simulink model "full_simulation_split_hil_new_connection"  (Simulink 7.9)
settings: Solver=ode1  StartTime=0  StopTime=10  FixedStep=Ts  RelTol=1e-8
values from neighbouring files (symbols this model uses):
  A_fx = 2e-2 * 0.4    (= 0.008)    [QR_DI_Init.m]    (also in quadro_cascade_disturbance_wo_wind.m)
  A_fy = A_fx    (= 0.008)    [QR_DI_Init.m]    (also in quadro_cascade_disturbance_wo_wind.m)
  A_fz = 2 * A_fx    (= 0.016)    [QR_DI_Init.m]    (also in quadro_cascade_disturbance_wo_wind.m)
  Bias_Phi = -0.0088    [QR_DI_Init.m]    (also in Reference_Calibration.m = mean(Phi))
  Bias_Theta = 0.022    [QR_DI_Init.m]    (also in Reference_Calibration.m = mean(Theta))
  command_on = 1    [QR_DI_Init.m]    (also in quadro_cascade_disturbance_wo_wind.m)
  cw_x = 1.05    [QR_DI_Init.m]    (also in quadro_cascade_disturbance_wo_wind.m)
  cw_y = cw_x    (= 1.05)    [QR_DI_Init.m]    (also in quadro_cascade_disturbance_wo_wind.m)
  cw_z = 1.05    [QR_DI_Init.m]    (also in quadro_cascade_disturbance_wo_wind.m)
  deltaTm = 0.2    [QR_DI_Init.m]    (also in quadro_cascade_disturbance_wo_wind.m)
  den_psi_ref = poly( ones(1,2) * -1 * T_psi_ref)    [QR_DI_Init.m]    (also in quadro_cascade_disturbance_wo_wind.m)
  den_x_ref = poly( ones(1,4) * -1 * T_x_ref)    [QR_DI_Init.m]    (also in quadro_cascade_disturbance_wo_wind.m)
  den_y_ref = poly( ones(1,4) * -1 * T_y_ref)    [QR_DI_Init.m]    (also in quadro_cascade_disturbance_wo_wind.m)
  den_z_ref = poly( ones(1,4) * -1 * T_z_ref)    [QR_DI_Init.m]    (also in quadro_cascade_disturbance_wo_wind.m)
  drot = 0.0117    [QR_DI_Init.m]    (also in quadro_cascade_disturbance_wo_wind.m = 0.2)
  dtran = 0.01    [QR_DI_Init.m]    (also in quadro_cascade_disturbance_wo_wind.m = 0.003)
  Fz_gain = 1 + 0.05*rand(1)    [QR_DI_Init.m]    (also in quadro_cascade_disturbance_wo_wind.m)
  Fz_lo = - 1.2 * m * g    (= -3.5316)    [QR_DI_Init.m]    (also in quadro_cascade_disturbance_wo_wind.m = -4.1202)
  Fz_up = 0    [QR_DI_Init.m]    (also in quadro_cascade_disturbance_wo_wind.m)
  g = 9.81    [QR_DI_Init.m]    (also in quadro_cascade_disturbance_wo_wind.m)
  Iq = [I_xx 0 0 ; 0 I_yy 0 ; 0 0 I_zz ]    [QR_DI_Init.m]    (also in quadro_cascade_disturbance_wo_wind.m = [0.0605 0 0; 0 0.0605 0; 0 0 0.018])
  K_err = old(:,2:end)    [QR_DI_Init.m]    (also in quadro_cascade_disturbance_wo_wind.m)
  K_Mot_Force = 0.3512    [QR_DI_Init.m]    (also in quadro_cascade_disturbance_wo_wind.m)
  K_Mot_Torque = 0.013    [QR_DI_Init.m]    (also in quadro_cascade_disturbance_wo_wind.m = 0.0013)
  l = 0.25    [QR_DI_Init.m]    (also in quadro_cascade_disturbance_wo_wind.m = 0.2775)
  m = 0.30    (= 0.3)    [QR_DI_Init.m]    (also in quadro_cascade_disturbance_wo_wind.m)
  m_real = m * ( 1 + 0.05*rand(1))    [QR_DI_Init.m]    (also in quadro_cascade_disturbance_wo_wind.m)
  Mm = 0.0    (= 0)    [QR_DI_Init.m]    (also in quadro_cascade_disturbance_wo_wind.m = 0.5)
  Mx_lo = - Mx_up    (= -0.2)    [QR_DI_Init.m]    (also in quadro_cascade_disturbance_wo_wind.m)
  Mx_up = 0.20    (= 0.2)    [QR_DI_Init.m]    (also in quadro_cascade_disturbance_wo_wind.m)
  My_lo = - My_up    (= -0.2)    [QR_DI_Init.m]    (also in quadro_cascade_disturbance_wo_wind.m)
  My_up = 0.20    (= 0.2)    [QR_DI_Init.m]    (also in quadro_cascade_disturbance_wo_wind.m)
  Mz_lo = - Mz_up    (= -0.02)    [QR_DI_Init.m]    (also in quadro_cascade_disturbance_wo_wind.m = -0.002)
  Mz_up = 0.02    [QR_DI_Init.m]    (also in quadro_cascade_disturbance_wo_wind.m = 0.002)
  phase_wind_z = 0    [QR_DI_Init.m]    (also in quadro_cascade_disturbance_wo_wind.m)
  psi_p_lim = 10*pi/180    (= 0.174532925199)    [QR_DI_Init.m]    (also in quadro_cascade_disturbance_wo_wind.m = 5)
  PWM_MAX = 200    [QR_DI_Init.m]    (also in quadro_cascade_disturbance_wo_wind.m)
  rho_air = 1.2041    [QR_DI_Init.m]    (also in quadro_cascade_disturbance_wo_wind.m)
  sample_time_noise_psi = 0.1    [QR_DI_Init.m]
  sample_time_noise_x = 0.2    [QR_DI_Init.m]
  sample_time_noise_y = 0.2    [QR_DI_Init.m]
  sample_time_noise_z = 0.1    [QR_DI_Init.m]
  seed_psi = seedvector(7)    [QR_DI_Init.m]
  seed_x = seedvector(1)    [QR_DI_Init.m]    (also in quadro_cascade_disturbance_wo_wind.m)
  seed_xp = seedvector(4)    [QR_DI_Init.m]    (also in quadro_cascade_disturbance_wo_wind.m)
  seed_y = seedvector(2)    [QR_DI_Init.m]    (also in quadro_cascade_disturbance_wo_wind.m)
  seed_yp = seedvector(5)    [QR_DI_Init.m]    (also in quadro_cascade_disturbance_wo_wind.m)
  seed_z = seedvector(3)    [QR_DI_Init.m]    (also in quadro_cascade_disturbance_wo_wind.m)
  seed_zp = seedvector(6)    [QR_DI_Init.m]    (also in quadro_cascade_disturbance_wo_wind.m)
  std_dev_psi = 1 * pi/180 * Noise_on    (= 0)    [QR_DI_Init.m]
  std_dev_x = 1e-1 * Noise_on    (= 0)    [QR_DI_Init.m]
  std_dev_xp = 0.03 * Noise_on    (= 0)    [QR_DI_Init.m]
  std_dev_y = 1e-1 * Noise_on    (= 0)    [QR_DI_Init.m]
  std_dev_yp = 0.03 * Noise_on    (= 0)    [QR_DI_Init.m]
  std_dev_z = 0.03 * Noise_on    (= 0)    [QR_DI_Init.m]
  std_dev_zp = 0.03 * Noise_on    (= 0)    [QR_DI_Init.m]
  T_refalt = 0.01    [QR_DI_Init.m]    (also in quadro_cascade_disturbance_wo_wind.m)
  T_wind_z = 24    [QR_DI_Init.m]    (also in quadro_cascade_disturbance_wo_wind.m)
  Tm = 10    [QR_DI_Init.m]    (also in quadro_cascade_disturbance_wo_wind.m)
  Ts = 1e-2    (= 0.01)    [QR_DI_Init.m]    (also in quadro_cascade_disturbance_wo_wind.m)
  v_wind_max_z = 2    [QR_DI_Init.m]    (also in quadro_cascade_disturbance_wo_wind.m)
  wind_on = 0    [QR_DI_Init.m]    (also in quadro_cascade_disturbance_wo_wind.m)
  x_p_lim = 1.5    [QR_DI_Init.m]    (also in quadro_cascade_disturbance_wo_wind.m = 5)
  y_p_lim = 1.5    [QR_DI_Init.m]    (also in quadro_cascade_disturbance_wo_wind.m = 5)
  z_p_lim = 1    [QR_DI_Init.m]    (also in quadro_cascade_disturbance_wo_wind.m = 1.5)
undefined symbols (not defined in the file or in its folder): T_wind_fine, v_wind_x_fine, v_wind_y_fine
libraries: simulink x5, dspsigops x4, Ports x4, aerolibtransform2 x3, dspmtrx3 x1, aerolibutil x1
(part 1 of 6)
settings Model: Creator=Richard  LastModifiedBy=uav  SimulationMode=accelerator  ExtModeTrigDuration=100
settings OptimizationCC: InitFltsAndDblsToZero=on
settings DebuggingCC: FcnCallInpInsideContextMsg=Use local settings  StrictBusMsg=Warning
settings HardwareCC: ProdIntDivRoundTo=Zero  ProdEndianess=LittleEndian  ProdHWDeviceType=Intel->x86/Pentium  TargetBitPerLong=64  TargetBitPerPointer=64  TargetEndianess=LittleEndian  TargetWordSize=64  TargetHWDeviceType=MATLAB Host  ProdEqTarget=off
settings RTWCC: SystemTargetFile=orocos.tlc  TemplateMakefile=orocos.tmf  Description=Linux Orocos Target  RTWVerbose=off  ProcessScript=orocos_make_rtw_hook
settings CodeAppCC: GenerateComments=off  MaxIdLength=128  SimulinkBlockComments=off
settings STFCustomTargetCC: CodeReplacementLibrary=ANSI_C  ModelReferenceCompliant=off  GeneratePreprocessorConditionals=Disable all  MatFileLogging=on  SystemTargetFile=orocos.tlc

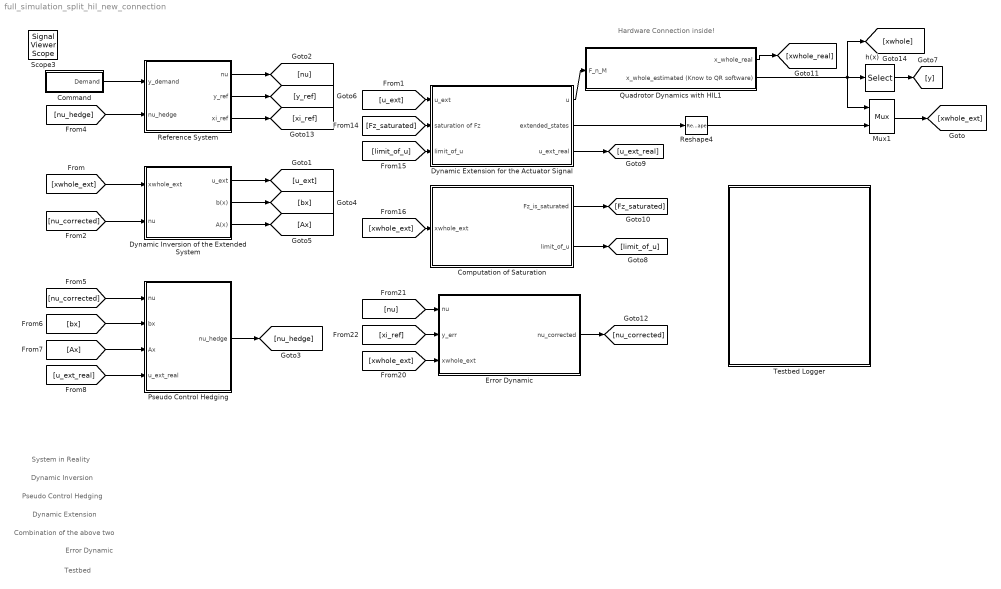
== system full_simulation_split_hil_new_connection ==
  note: System in Reality
  note: Dynamic Extension
  note: Dynamic Inversion
  note: Pseudo Control Hedging
  note: Combination of the above two
  note: Error Dynamic
  note: Testbed
  note: Hardware Connection inside!
  Command : Subsystem
  Computation of Saturation : Subsystem
  Dynamic Extension for the Actuator Signal : Subsystem
  Dynamic Inversion of the Extended System : Subsystem
  Error Dynamic : Subsystem
  Mux1 : Mux  Inputs=2
  Pseudo Control Hedging : Subsystem
  Quadrotor Dynamics with HIL1 : Subsystem
  Reference System : Subsystem
  Reshape4 : Reshape  OutputDimensionality=Column vector (2-D)  OutputDimensions=[1:3]
  Testbed Logger : Subsystem
  h(x) : Selector  InputPortWidth=12  IndexOptions=Index vector (dialog)  Indices=[1 2 3 9]  OutputSizes=1
  Scope3 : SignalViewerScope  IOType=viewer  NumInputPorts=4  RefreshTime=0.035000
  wires:
  Reference System/1(nu) -> [nu]
  Dynamic Extension for the Actuator Signal/1(u) -> Quadrotor Dynamics with HIL1/1(F_n_M)
  Quadrotor Dynamics with HIL1/2(x_whole_estimated (Know to QR software)) -> h(x)/1, [xwhole], Mux1/1
  Dynamic Extension for the Actuator Signal/2(extended_states) -> Reshape4/1
  Dynamic Inversion of the Extended System/1(u_ext) -> [u_ext]
  Mux1/1 -> [xwhole_ext]
  [u_ext] -> Dynamic Extension for the Actuator Signal/1(u_ext)
  Reshape4/1 -> Mux1/2
  h(x)/1 -> [y]
  [nu_hedge] -> Reference System/2(nu_hedge)
  [xwhole_ext] -> Dynamic Inversion of the Extended System/1(xwhole_ext)
  [nu_corrected] -> Dynamic Inversion of the Extended System/2(nu)
  Dynamic Inversion of the Extended System/2(b(x)) -> [bx]
  Dynamic Inversion of the Extended System/3(A(x)) -> [Ax]
  [nu_corrected] -> Pseudo Control Hedging/1(nu)
  [bx] -> Pseudo Control Hedging/2(bx)
  [Ax] -> Pseudo Control Hedging/3(Ax)
  [u_ext_real] -> Pseudo Control Hedging/4(u_ext_real)
  Reference System/2(y_ref) -> [y_ref]
  Pseudo Control Hedging/1(nu_hedge) -> [nu_hedge]
  [Fz_saturated] -> Dynamic Extension for the Actuator Signal/2(saturation of Fz)
  Dynamic Extension for the Actuator Signal/3(u_ext_real) -> [u_ext_real]
  Computation of Saturation/2(limit_of_u) -> [limit_of_u]
  [limit_of_u] -> Dynamic Extension for the Actuator Signal/3(limit_of_u)
  [xwhole_ext] -> Computation of Saturation/1(xwhole_ext)
  Computation of Saturation/1(Fz_is_saturated) -> [Fz_saturated]
  Reference System/3(xi_ref) -> [xi_ref]
  [nu] -> Error Dynamic/1(nu)
  [xi_ref] -> Error Dynamic/2(y_err)
  [xwhole_ext] -> Error Dynamic/3(xwhole_ext)
  Error Dynamic/1(nu_corrected) -> [nu_corrected]
  Command/1(Demand) -> Reference System/1(y_demand)
  Quadrotor Dynamics with HIL1/1(x_whole_real) -> [xwhole_real]

== system full_simulation_split_hil_new_connection/Command ==
  CommandOn : Gain  Gain=command_on
  From Workspace : FromWorkspace  VariableName=Mission_Outdoor_steps  SampleTime=0  Interpolate=off  OutputAfterFinalValue=Holding final value
  From Workspace1 : FromWorkspace  VariableName=Mission_Indoor_steps  SampleTime=0  Interpolate=off  OutputAfterFinalValue=Holding final value
  Step 1 : Step  Time=75  Before=zeros(1,4)  After=[25 15 -25 20*pi/180]*1  SampleTime=0
  Step 2 : Step  Time=100  Before=zeros(1,4)  After=[-24 -24 20 -40*pi/180]*1  SampleTime=0
  Step 3 : Step  Time=15  Before=zeros(1,4)  After=[50 50 50 0]*1  SampleTime=0
  Sum2 : Sum  Inputs=2
  Demand : Outport
  wires:
  Sum2/1 -> CommandOn/1
  CommandOn/1 -> Demand/1
  From Workspace/1 -> Sum2/1

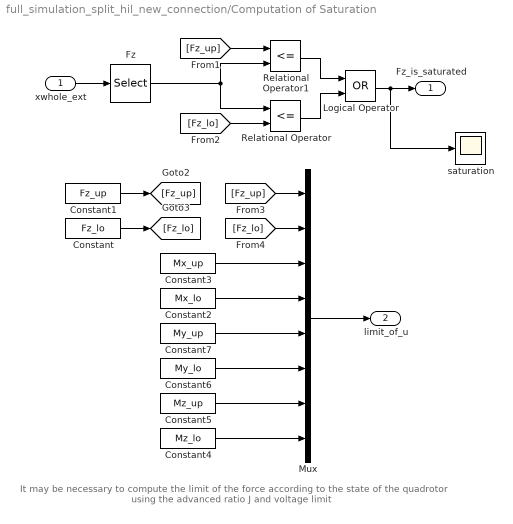
== system full_simulation_split_hil_new_connection/Computation of Saturation ==
  note: It may be necessary to compute the limit of the force according to
      | the state of the quadrotor using the advanced ratio J and voltage limit
  xwhole_ext : Inport
  Constant : Constant  Value=Fz_lo
  Constant1 : Constant  Value=Fz_up
  Constant2 : Constant  Value=Mx_lo
  Constant3 : Constant  Value=Mx_up
  Constant4 : Constant  Value=Mz_lo
  Constant5 : Constant  Value=Mz_up
  Constant6 : Constant  Value=My_lo
  Constant7 : Constant  Value=My_up
  Fz : Selector  InputPortWidth=14  IndexOptions=Index vector (dialog)  Indices=[13]  OutputSizes=1
  Logical Operator : Logic  Operator=OR  AllPortsSameDT=off  OutDataTypeStr=boolean
  Mux : Mux  Inputs=8
  Relational Operator : RelationalOperator  Operator=<=  OutDataTypeStr=boolean
  Relational Operator1 : RelationalOperator  Operator=<=  OutDataTypeStr=boolean
  saturation : Scope
      settings: YMin=-27.5  YMax=27.5  SaveName=ScopeData11
  Fz_is_saturated : Outport
  limit_of_u : Outport  Port=2
  wires:
  xwhole_ext/1 -> Fz/1
  [Fz_up] -> Mux/1
  [Fz_lo] -> Mux/2
  Constant1/1 -> [Fz_up]
  Constant/1 -> [Fz_lo]
  Constant3/1 -> Mux/3
  Constant4/1 -> Mux/8
  Constant2/1 -> Mux/4
  Constant7/1 -> Mux/5
  Constant6/1 -> Mux/6
  Constant5/1 -> Mux/7
  [Fz_up] -> Relational Operator1/1
  Relational Operator1/1 -> Logical Operator/1
  Relational Operator/1 -> Logical Operator/2
  Logical Operator/1 -> Fz_is_saturated/1, saturation/1
  Mux/1 -> limit_of_u/1
  [Fz_lo] -> Relational Operator/2
  Fz/1 -> Relational Operator1/2, Relational Operator/1

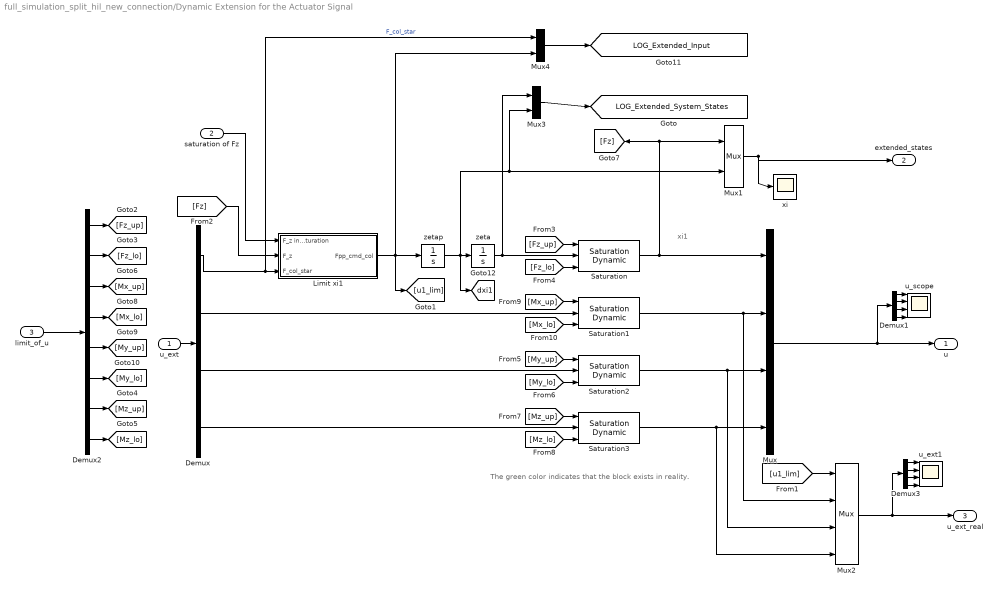
== system full_simulation_split_hil_new_connection/Dynamic Extension for the Actuator Signal ==
  note: xi1
  note: The green color indicates that the
      | block exists in reality.
  u_ext : Inport
  saturation of Fz : Inport  Port=2
  limit_of_u : Inport  Port=3
  Demux : Demux
  Demux1 : Demux
  Demux2 : Demux  Outputs=8
  Demux3 : Demux
  Limit xi1 : Subsystem
  Mux : Mux
  Mux1 : Mux  Inputs=2
  Mux2 : Mux
  Mux3 : Mux  Inputs=2
  Mux4 : Mux  Inputs=2
  Saturation{,1..3} (4 alike) : simulink/Discontinuities/Saturation Dynamic  OutMin=[]  OutMax=[]  OutDataTypeStr=Inherit: Same as second input  OutDataType=sfix(16)  OutScaling=2^-10  DoSatur=off
  u_ext1 : Scope  NumInputPorts=4
      settings: TimeRange=1  YMin=0~0~0~-5  YMax=1~1~1~5  SaveName=ScopeData9
  u_scope : Scope  NumInputPorts=4
      settings: TimeRange=40  YMin=8~-6~-15~-8  YMax=20~8~10~4  SaveName=ScopeData12
  xi : Scope
      settings: YMin=-27.5  YMax=27.5  SaveName=ScopeData7
  zeta : Integrator
  zetap : Integrator
  u : Outport
  extended_states : Outport  Port=2
  u_ext_real : Outport  Port=3
  tag scope: LOG_Extended_Input=global, LOG_Extended_System_States=global, dxi1=global
  wires:
  u_ext/1 -> Demux/1
  Demux/2 -> Saturation1/2
  Demux/3 -> Saturation2/2
  Demux/4 -> Saturation3/2
  zeta/1 -> Saturation/2, Mux3/1
  Mux1/1 -> extended_states/1, xi/1
  Demux1/1 -> u_scope/1
  Demux1/2 -> u_scope/2
  Demux1/3 -> u_scope/3
  Demux1/4 -> u_scope/4
  saturation of Fz/1 -> Limit xi1/1(F_z in saturation)
  Mux2/1 -> u_ext_real/1, Demux3/1
  Demux/1 -> Limit xi1/3(F_col_star), Mux4/1  "F_col_star"
  [Fz] -> Limit xi1/2(F_z)
  Saturation/1 -> Mux/1, Mux1/1, [Fz]
  Saturation1/1 -> Mux/2, Mux2/2
  Saturation2/1 -> Mux/3, Mux2/3
  Saturation3/1 -> Mux/4, Mux2/4
  Mux/1 -> u/1, Demux1/1
  [u1_lim] -> Mux2/1
  [Fz_up] -> Saturation/1
  [Fz_lo] -> Saturation/3
  [Mz_up] -> Saturation3/1
  [Mz_lo] -> Saturation3/3
  [Mx_up] -> Saturation1/1
  [Mx_lo] -> Saturation1/3
  [My_up] -> Saturation2/1
  [My_lo] -> Saturation2/3
  Demux2/1 -> [Fz_up]
  Demux2/2 -> [Fz_lo]
  Demux2/3 -> [Mx_up]
  Demux2/4 -> [Mx_lo]
  Demux2/5 -> [My_up]
  Demux2/6 -> [My_lo]
  Demux2/7 -> [Mz_up]
  Demux2/8 -> [Mz_lo]
  limit_of_u/1 -> Demux2/1
  Demux3/1 -> u_ext1/1
  Demux3/2 -> u_ext1/2
  Demux3/3 -> u_ext1/3
  Demux3/4 -> u_ext1/4
  Limit xi1/1(Fpp_cmd_col) -> [u1_lim], zetap/1, Mux4/2
  zetap/1 -> [dxi1], zeta/1, Mux1/2, Mux3/2
  Mux3/1 -> [LOG_Extended_System_States]
  Mux4/1 -> [LOG_Extended_Input]

== system full_simulation_split_hil_new_connection/Dynamic Inversion of the Extended System ==
  xwhole_ext : Inport
  nu : Inport  Port=2
  Add2 : Sum
  Ber. alpha(x) : Subsystem
  Ber. beta(x) : Subsystem
  Divide1 : Product  Inputs=**  Multiplication=Matrix(*)
  bx SH : Subsystem  mask{m=m, Iq=Iq, dtran=dtran, drot=drot}
      mask prompts: m "Mass"; Iq "Inertia"; dtran "Translational Damping Constan"; drot "Rotational Damping Constant"
  bx1 : Subsystem  mask{m=m, Iq=Iq, dtran=dtran, drot=drot}
      mask prompts: m "Mass"; Iq "Inertia"; dtran "Translational Damping Constan"; drot "Rotational Damping Constant"
  invAx SH : Subsystem  mask{m=m, Iq=Iq, dtran=dtran, drot=drot}
      mask prompts: m "Mass"; Iq "Inertia"; dtran "Translational Damping Constan"; drot "Rotational Damping Constant"
  invAx1 : Subsystem  mask{m=m, Iq=Iq, dtran=dtran, drot=drot}
      mask prompts: m "Mass"; Iq "Inertia"; dtran "Translational Damping Constan"; drot "Rotational Damping Constant"
  u_ext : Outport
  b(x) : Outport  Port=2
  A(x) : Outport  Port=3
  wires:
  Divide1/1 -> Add2/1
  Ber. alpha(x)/1(alpha (x)) -> Add2/2
  Ber. beta(x)/1(beta (x)) -> Divide1/1
  nu/1 -> Divide1/2
  bx SH/1(bx) -> Ber. alpha(x)/2(b (x)), b(x)/1  "b(x)"
  xwhole_ext/1 -> invAx SH/1(xwhole_ext), bx SH/1(xwhole_ext)
  invAx SH/1(invAx) -> Ber. beta(x)/1(A_inv(x)), Ber. alpha(x)/1(A_inv(x))
  Add2/1 -> u_ext/1
  invAx SH/2(A(x)) -> A(x)/1

== system full_simulation_split_hil_new_connection/Error Dynamic ==
  nu : Inport
  y_err : Inport  Port=2
  xwhole_ext : Inport  Port=3
  K_err*u : Gain  Gain=K_err  Multiplication=Matrix(K*u) (u vector)
  Sum1 : Sum  Inputs=+-|
  Sum2 : Sum  Inputs=++|
  add inegratorl1 : Subsystem
  add inegratorl2 : Subsystem
  coordinate transformation1 : Subsystem  mask{m=m, Iq=Iq, dtran=dtran, drot=drot}
      mask prompts: m "Mass"; Iq "Inertia"; dtran "Translational Damping Constan"; drot "Rotational Damping Constant"
  nu_corrected : Outport
  tag scope: LOG_External_Dynamics_State_Vector=global, LOG_Reference_Input=global
  wires:
  coordinate transformation1/1(xi) -> add inegratorl1/1(In1), [LOG_External_Dynamics_State_Vector]
  Sum1/1 -> K_err*u/1
  y_err/1 -> add inegratorl2/1(In1)
  nu/1 -> Sum2/1
  Sum2/1 -> nu_corrected/1, [LOG_Reference_Input]
  xwhole_ext/1 -> coordinate transformation1/1(xwhole_ext)
  K_err*u/1 -> Sum2/2
  add inegratorl1/1(Out1) -> Sum1/2
  add inegratorl2/1(Out1) -> Sum1/1

== system full_simulation_split_hil_new_connection/Pseudo Control Hedging ==
  nu : Inport
  bx : Inport  Port=2
  Ax : Inport  Port=3
  u_ext_real : Inport  Port=4
  Add4 : Sum  Inputs=+-
  Divide4 : Product  Inputs=**  Multiplication=Matrix(*)
  nu_hat : Sum
  nu_hedge : Outport
  tag scope: LOG_Estimated_Sys_Output=global, LOG_Hedge_Signal_Vector=global
  wires:
  Divide4/1 -> nu_hat/2
  nu_hat/1 -> Add4/2, [LOG_Estimated_Sys_Output]
  nu/1 -> Add4/1
  Add4/1 -> nu_hedge/1, [LOG_Hedge_Signal_Vector]
  bx/1 -> nu_hat/1
  Ax/1 -> Divide4/1
  u_ext_real/1 -> Divide4/2

== system full_simulation_split_hil_new_connection/Quadrotor Dynamics with HIL1 ==
  note: Real: simulated reality, no noise
      | IMU: IMU from QR
  F_n_M : Inport
  Data Fusion : Subsystem
  Fz_cmd : Selector  InputPortWidth=4  IndexOptions=Index vector (dialog)  Indices=[1]  OutputSizes=1
  M_cmd : Selector  InputPortWidth=4  IndexOptions=Index vector (dialog)  Indices=[2:4]  OutputSizes=1
  Sensor Model : Subsystem
  Simulated Reality : Subsystem
  x_whole_real : Outport
  x_whole_estimated (Know to QR software) : Outport  Port=2
  tag scope: LOG_Input_Vector=global, LOG_State_Vector=global
  wires:
  M_cmd/1 -> Simulated Reality/2(M_b)
  Fz_cmd/1 -> Simulated Reality/1(F_z(b))
  Simulated Reality/2(x_whole_real) -> x_whole_real/1, Sensor Model/1(x_whole_real)
  Data Fusion/1(x_whole_estimated) -> x_whole_estimated (Know to QR software)/1, [LOG_State_Vector]
  Sensor Model/3(Yaw Angle) -> Data Fusion/4(Psi)  "Psi"
  Sensor Model/1(x_vec (Position)) -> Data Fusion/2(x_Vector)
  Sensor Model/2(xp_vec (Velocity)) -> Data Fusion/3(xp_Vector)
  Simulated Reality/1("x_angular_IMU (x_Euler, Omega)") -> Data Fusion/1("x_Euler, Omega")
  F_n_M/1 -> Fz_cmd/1, M_cmd/1, [LOG_Input_Vector]

== system full_simulation_split_hil_new_connection/Reference System ==
  y_demand : Inport
  nu_hedge : Inport  Port=2
  Rate Limiter : RateLimiter  RisingSlewLimit=[ x_p_lim y_p_lim z_p_lim psi_p_lim ]  FallingSlewLimit=- [ x_p_lim y_p_lim z_p_lim psi_p_lim ]  SampleTimeMode=inherited
  Reference System : Subsystem
  nu : Outport
  y_ref : Outport  Port=2
  xi_ref : Outport  Port=3
  tag scope: LOG_Demand=global, LOG_Reference_Sys_Output=global
  wires:
  y_demand/1 -> Rate Limiter/1, [LOG_Demand]
  Reference System/1(nu) -> nu/1, [LOG_Reference_Sys_Output]
  Reference System/2(y_ref) -> y_ref/1
  Reference System/3(xi_ref) -> xi_ref/1
  nu_hedge/1 -> Reference System/2(nu_hedge)
  Rate Limiter/1 -> Reference System/1(command)

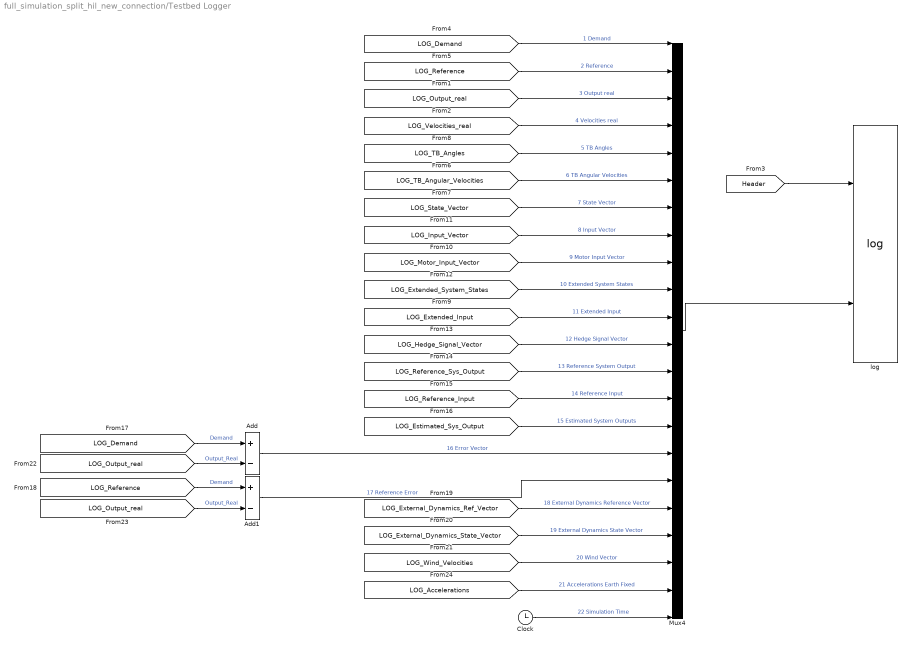
== system full_simulation_split_hil_new_connection/Testbed Logger ==
  Add : Sum  Inputs=+-
  Add1 : Sum  Inputs=+-
  Clock : Clock
  Mux4 : Mux  Inputs=22
  log : Ports/log
  wires:
  [Header] -> log/1
  Mux4/1 -> log/2
  [LOG_Demand] -> Mux4/1  "1 Demand"
  [LOG_Reference] -> Mux4/2  "2 Reference"
  [LOG_Output_real] -> Mux4/3  "3 Output real"
  [LOG_Velocities_real] -> Mux4/4  "4 Velocities real"
  [LOG_TB_Angles] -> Mux4/5  "5 TB Angles"
  [LOG_TB_Angular_Velocities] -> Mux4/6  "6 TB Angular Velocities"
  [LOG_State_Vector] -> Mux4/7  "7 State Vector"
  [LOG_Input_Vector] -> Mux4/8  "8 Input Vector"
  [LOG_Motor_Input_Vector] -> Mux4/9  "9 Motor Input Vector"
  [LOG_Extended_System_States] -> Mux4/10  "10 Extended System States"
  [LOG_Extended_Input] -> Mux4/11  "11 Extended Input"
  [LOG_Hedge_Signal_Vector] -> Mux4/12  "12 Hedge Signal Vector"
  [LOG_Reference_Sys_Output] -> Mux4/13  "13 Reference System Output"
  [LOG_Reference_Input] -> Mux4/14  "14 Reference Input"
  [LOG_Estimated_Sys_Output] -> Mux4/15  "15 Estimated System Outputs"
  Add/1 -> Mux4/16  "16 Error Vector"
  Add1/1 -> Mux4/17  "17 Reference Error"
  [LOG_External_Dynamics_Ref_Vector] -> Mux4/18  "18 External Dynamics Reference Vector"
  [LOG_External_Dynamics_State_Vector] -> Mux4/19  "19 External Dynamics State Vector"
  [LOG_Wind_Velocities] -> Mux4/20  "20 Wind Vector"
  [LOG_Demand] -> Add/1  "Demand"
  [LOG_Output_real] -> Add/2  "Output_Real"
  [LOG_Reference] -> Add1/1  "Demand"
  [LOG_Output_real] -> Add1/2  "Output_Real"
  [LOG_Accelerations] -> Mux4/21  "21 Accelerations Earth Fixed"
  Clock/1 -> Mux4/22  "22 Simulation Time"

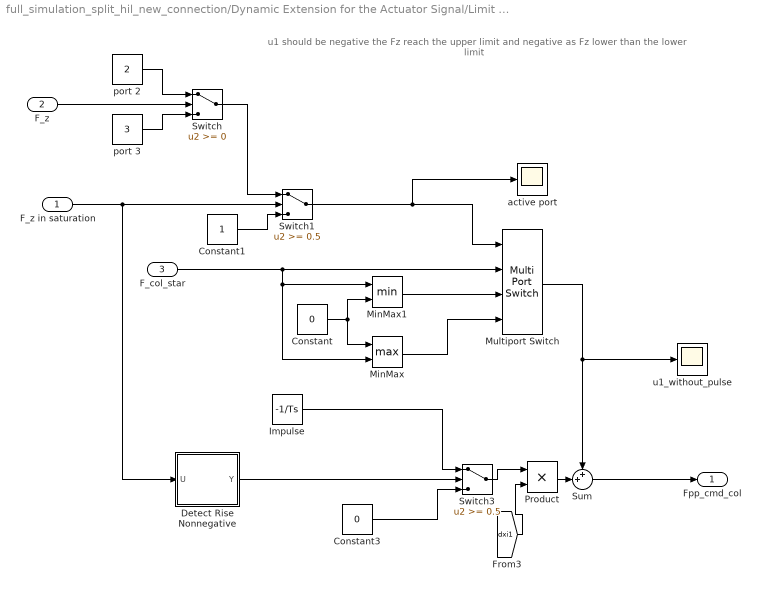
== system full_simulation_split_hil_new_connection/Dynamic Extension for the Actuator Signal/Limit xi1 ==
  note: u1 should be negative the Fz reach the upper limit and negative as Fz lower than the lower limit
  F_z in saturation : Inport
  F_z : Inport  Port=2
  F_col_star : Inport  Port=3
  Constant : Constant  Value=0
  Constant1 : Constant
  Constant3 : Constant  Value=0
  Detect Rise Nonnegative : Subsystem  AncestorBlock=|  mask(Detect Rise Nonnegative){vinit=0}
      | simulink/Logic and Bit
      | Operations/Detect Rise
      | Nonnegative
      mask prompts: vinit "Initial condition:"
      mask help: If the input is nonnegative and its previous value was strictly negative, then output TRUE, otherwise output FALSE. The initial condition determines the initial value of the boolean expression (U/z >= 0).
      mask init:
      | vinit=double(vinit);
      mask Display: fprintf('U >= 0\n&  NOT\nU/z >= 0')
  Impulse : Constant  Value=-1/Ts
  MinMax : MinMax  Function=max  Inputs=2
  MinMax1 : MinMax  Inputs=2
  Multiport Switch : MultiPortSwitch  zeroidx=off
  Product : Product  RndMeth=Zero
  Sum : Sum  Inputs=++|
  Switch : Switch
  Switch1 : Switch  Threshold=0.5
  Switch3 : Switch  Threshold=0.5
  active port : Scope
      settings: YMin=1  YMax=2  SaveName=ScopeData10
  port 2 : Constant  Value=2
  port 3 : Constant  Value=3
  u1_without_pulse : Scope
      settings: YMin=-3  YMax=14  SaveName=ScopeData18
  Fpp_cmd_col : Outport
  wires:
  F_col_star/1 -> Multiport Switch/2, MinMax1/1, MinMax/2
  MinMax1/1 -> Multiport Switch/3
  MinMax/1 -> Multiport Switch/4
  Constant/1 -> MinMax1/2, MinMax/1
  Multiport Switch/1 -> Sum/1, u1_without_pulse/1
  port 2/1 -> Switch/1
  port 3/1 -> Switch/3
  F_z/1 -> Switch/2
  Switch/1 -> Switch1/1
  F_z in saturation/1 -> Switch1/2, Detect Rise Nonnegative/1(U)
  Constant1/1 -> Switch1/3
  Switch1/1 -> Multiport Switch/1, active port/1
  Impulse/1 -> Switch3/1
  Detect Rise Nonnegative/1(Y) -> Switch3/2
  Sum/1 -> Fpp_cmd_col/1
  Constant3/1 -> Switch3/3
  Product/1 -> Sum/2
  Switch3/1 -> Product/1
  [dxi1] -> Product/2

== system full_simulation_split_hil_new_connection/Dynamic Inversion of the Extended System/Ber. alpha(x) ==
  A_inv(x) : Inport
  b (x) : Inport  Port=2
  Divide2 : Product  Inputs=**  Multiplication=Matrix(*)
  Gain2 : Gain  Gain=-1
  alpha (x) : Outport
  wires:
  Divide2/1 -> Gain2/1  "alpha (x)"
  Gain2/1 -> alpha (x)/1
  A_inv(x)/1 -> Divide2/1
  b (x)/1 -> Divide2/2

== system full_simulation_split_hil_new_connection/Dynamic Inversion of the Extended System/Ber. beta(x) ==
  A_inv(x) : Inport
  beta (x) : Outport
  wires:
  A_inv(x)/1 -> beta (x)/1

== system full_simulation_split_hil_new_connection/Dynamic Inversion of the Extended System/bx SH ==
  xwhole_ext : Inport
  Constant3 : Constant  Value=dtran
  Constant4 : Constant  Value=drot
  Embedded MATLAB Function1 : MATLAB Function  TreatAsAtomicUnit=on
  inertia1 : Constant  Value=Iq
  m : Constant  Value=m
  bx : Outport
  wires:
  Constant3/1 -> Embedded MATLAB Function1/4(dtran)
  m/1 -> Embedded MATLAB Function1/2(m_in)
  inertia1/1 -> Embedded MATLAB Function1/3(I)
  Constant4/1 -> Embedded MATLAB Function1/5(drot)
  xwhole_ext/1 -> Embedded MATLAB Function1/1(xwhole_ext)
  Embedded MATLAB Function1/1(bx) -> bx/1

== system full_simulation_split_hil_new_connection/Dynamic Inversion of the Extended System/bx1 ==
  xwhole_ext : Inport
  Constant3 : Constant  Value=dtran
  Constant4 : Constant  Value=drot
  Embedded MATLAB Function1 : MATLAB Function  TreatAsAtomicUnit=on
  inertia1 : Constant  Value=Iq
  m : Constant  Value=m
  bx : Outport
  wires:
  Constant3/1 -> Embedded MATLAB Function1/4(dtran)
  m/1 -> Embedded MATLAB Function1/2(m_in)
  inertia1/1 -> Embedded MATLAB Function1/3(I)
  Constant4/1 -> Embedded MATLAB Function1/5(drot)
  xwhole_ext/1 -> Embedded MATLAB Function1/1(xwhole_ext)
  Embedded MATLAB Function1/1(bx) -> bx/1

== system full_simulation_split_hil_new_connection/Dynamic Inversion of the Extended System/invAx SH ==
  xwhole_ext : Inport
  Constant3 : Constant  Value=dtran
  Constant4 : Constant  Value=drot
  Embedded MATLAB Function : MATLAB Function  TreatAsAtomicUnit=on
  inertia1 : Constant  Value=Iq
  m : Constant  Value=m
  invAx : Outport
  A(x) : Outport  Port=2
  wires:
  Embedded MATLAB Function/2(Ax) -> A(x)/1
  Embedded MATLAB Function/1(invAx) -> invAx/1
  xwhole_ext/1 -> Embedded MATLAB Function/1(xwhole_ext)
  Constant4/1 -> Embedded MATLAB Function/5(drot)
  Constant3/1 -> Embedded MATLAB Function/4(dtran)
  inertia1/1 -> Embedded MATLAB Function/3(I)
  m/1 -> Embedded MATLAB Function/2(m)

== system full_simulation_split_hil_new_connection/Dynamic Inversion of the Extended System/invAx1 ==
  xwhole_ext : Inport
  Constant3 : Constant  Value=dtran
  Constant4 : Constant  Value=drot
  Embedded MATLAB Function : MATLAB Function  TreatAsAtomicUnit=on
  inertia1 : Constant  Value=Iq
  m : Constant  Value=m
  invAx : Outport
  A(x) : Outport  Port=2
  wires:
  Embedded MATLAB Function/2(Ax) -> A(x)/1
  Embedded MATLAB Function/1(invAx) -> invAx/1
  xwhole_ext/1 -> Embedded MATLAB Function/1(xwhole_ext)
  Constant4/1 -> Embedded MATLAB Function/5(drot)
  Constant3/1 -> Embedded MATLAB Function/4(dtran)
  inertia1/1 -> Embedded MATLAB Function/3(I)
  m/1 -> Embedded MATLAB Function/2(m)

== system full_simulation_split_hil_new_connection/Error Dynamic/add inegratorl1 ==
  In1 : Inport
  Demux : Demux  Outputs=14
  Integrator{,1..3} (4 alike) : Integrator
  Mux : Mux  Inputs=18
  Out1 : Outport
  wires:
  Integrator/1 -> Mux/1
  Demux/1 -> Mux/2, Integrator/1
  Demux/2 -> Mux/3
  Demux/3 -> Mux/4
  Demux/4 -> Mux/5
  Integrator1/1 -> Mux/6
  Demux/5 -> Mux/7, Integrator1/1
  Demux/6 -> Mux/8
  Demux/7 -> Mux/9
  Demux/8 -> Mux/10
  Integrator2/1 -> Mux/11
  Demux/9 -> Mux/12, Integrator2/1
  Demux/10 -> Mux/13
  Demux/11 -> Mux/14
  Demux/12 -> Mux/15
  Integrator3/1 -> Mux/16
  Demux/13 -> Mux/17, Integrator3/1
  Demux/14 -> Mux/18
  In1/1 -> Demux/1
  Mux/1 -> Out1/1

== system full_simulation_split_hil_new_connection/Error Dynamic/add inegratorl2 ==
  In1 : Inport
  Demux : Demux  Outputs=14
  Integrator{,1..3} (4 alike) : Integrator
  Mux : Mux  Inputs=18
  Out1 : Outport
  wires:
  Mux/1 -> Out1/1
  In1/1 -> Demux/1
  Demux/14 -> Mux/18
  Demux/13 -> Integrator3/1, Mux/17
  Integrator3/1 -> Mux/16
  Demux/12 -> Mux/15
  Demux/11 -> Mux/14
  Demux/10 -> Mux/13
  Demux/9 -> Integrator2/1, Mux/12
  Integrator2/1 -> Mux/11
  Demux/8 -> Mux/10
  Demux/7 -> Mux/9
  Demux/6 -> Mux/8
  Demux/5 -> Integrator1/1, Mux/7
  Integrator1/1 -> Mux/6
  Demux/4 -> Mux/5
  Demux/3 -> Mux/4
  Demux/2 -> Mux/3
  Demux/1 -> Integrator/1, Mux/2
  Integrator/1 -> Mux/1

== system full_simulation_split_hil_new_connection/Error Dynamic/coordinate transformation1 ==
  xwhole_ext : Inport
  Constant3 : Constant  Value=dtran
  Constant4 : Constant  Value=drot
  Embedded MATLAB Function : MATLAB Function  TreatAsAtomicUnit=on
  inertia1 : Constant  Value=Iq
  m : Constant  Value=m
  xi : Outport
  wires:
  m/1 -> Embedded MATLAB Function/2(m)
  inertia1/1 -> Embedded MATLAB Function/3(I)
  Constant3/1 -> Embedded MATLAB Function/4(dtran)
  Constant4/1 -> Embedded MATLAB Function/5(drot)
  xwhole_ext/1 -> Embedded MATLAB Function/1(xwhole_ext)
  Embedded MATLAB Function/1(xi) -> xi/1

== system full_simulation_split_hil_new_connection/Quadrotor Dynamics with HIL1/Data Fusion ==
  "x_Euler, Omega" : Inport
  x_Vector : Inport  Port=2
  xp_Vector : Inport  Port=3
  Psi : Inport  Port=4
  Mux : Mux  Inputs=2
  Mux1 : Mux
  Selector : Selector  InputPortWidth=6  IndexOptions=Index vector (dialog)  Indices=[1 2]  OutputSizes=1
  Selector1 : Selector  InputPortWidth=6  IndexOptions=Index vector (dialog)  Indices=[4:6]  OutputSizes=1
  x_whole_estimated : Outport
  wires:
  "x_Euler, Omega"/1 -> Selector1/1, Selector/1
  Selector/1 -> Mux/1  "Phi, Theta"
  Selector1/1 -> Mux1/4  "p,q,r"
  Mux/1 -> Mux1/3
  Psi/1 -> Mux/2
  x_Vector/1 -> Mux1/1
  xp_Vector/1 -> Mux1/2
  Mux1/1 -> x_whole_estimated/1

== system full_simulation_split_hil_new_connection/Quadrotor Dynamics with HIL1/Sensor Model ==
  x_whole_real : Inport
  Noise : Subsystem
  Noise1 : Subsystem
  Noise2 : Subsystem
  Position : Selector  InputPortWidth=12  IndexOptions=Index vector (dialog)  Indices=[1:3]  OutputSizes=1
  Velocity : Selector  InputPortWidth=12  IndexOptions=Index vector (dialog)  Indices=[4:6]  OutputSizes=1
  Yaw : Selector  InputPortWidth=12  IndexOptions=Index vector (dialog)  Indices=[9]  OutputSizes=1
  x_vec (Position) : Outport
  xp_vec (Velocity) : Outport  Port=2
  Yaw Angle : Outport  Port=3
  wires:
  Position/1 -> Noise/1(In1)
  Velocity/1 -> Noise1/1(In1)
  x_whole_real/1 -> Velocity/1, Position/1, Yaw/1
  Yaw/1 -> Noise2/1(In1)
  Noise/1(Out1) -> x_vec (Position)/1
  Noise1/1(Out1) -> xp_vec (Velocity)/1
  Noise2/1(Out1) -> Yaw Angle/1

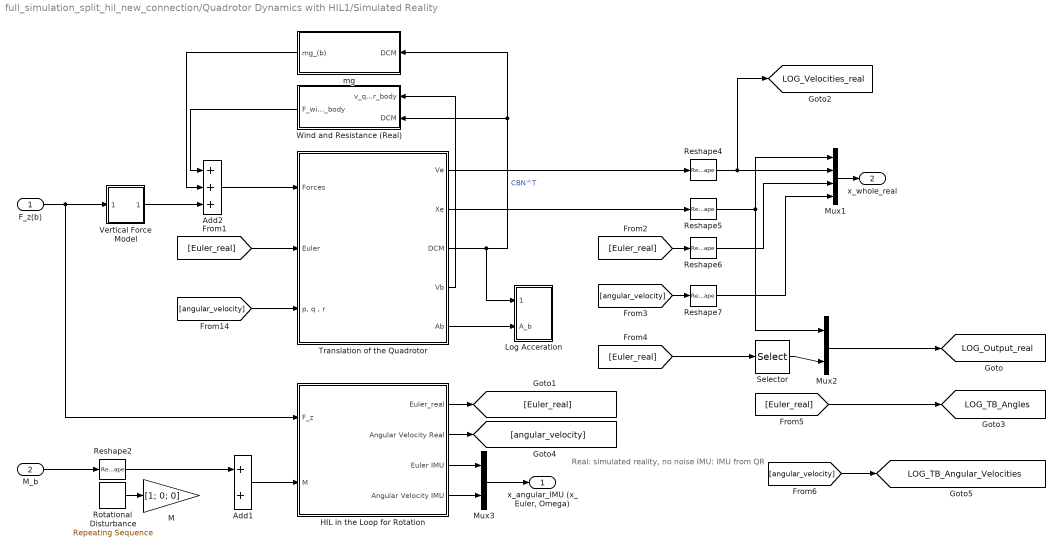
== system full_simulation_split_hil_new_connection/Quadrotor Dynamics with HIL1/Simulated Reality ==
  note: Real: simulated reality, no noise
      | IMU: IMU from QR
  F_z(b) : Inport
  M_b : Inport  Port=2
  Add1 : Sum  Inputs=2
  Add2 : Sum  Inputs=+++
  HIL in the Loop for Rotation : Subsystem
  Log Acceration : Subsystem
  M : Gain  Gain=[1; 0; 0]
  Mux1 : Mux
  Mux2 : Mux  Inputs=2
  Mux3 : Mux  Inputs=2
  Reshape2 : Reshape  OutputDimensions=[4:6]
  Reshape{4..7} (4 alike) : Reshape  OutputDimensionality=Column vector (2-D)  OutputDimensions=[1:3]
  Rotational Disturbance : simulink/Sources/Repeating Sequence  rep_seq_t=[0 Tm-deltaTm Tm]  rep_seq_y=[0 0 Mm]
  Selector : Selector  InputPortWidth=3  IndexOptions=Index vector (dialog)  Indices=[3]  OutputSizes=1
  Translation of the Quadrotor : Subsystem  mask{m=m_real}
      mask prompts: m "mass of the system"
  Vertical Force Model : Subsystem
  Wind and Resistance (Real) : Subsystem
  mg : Subsystem
  "x_angular_IMU (x_Euler, Omega)" : Outport
  x_whole_real : Outport  Port=2
  tag scope: LOG_Output_real=global, LOG_TB_Angles=global, LOG_TB_Angular_Velocities=global, LOG_Velocities_real=global
  wires:
  Translation of the Quadrotor/1(Ve) -> Reshape4/1
  F_z(b)/1 -> HIL in the Loop for Rotation/1(F_z), Vertical Force Model/1(F_z)
  Reshape4/1 -> Mux1/2, [LOG_Velocities_real]
  Reshape5/1 -> Mux1/1, Mux2/1
  Reshape6/1 -> Mux1/3
  Reshape7/1 -> Mux1/4
  Add2/1 -> Translation of the Quadrotor/1(Forces)
  Vertical Force Model/1(F_b) -> Add2/3
  Translation of the Quadrotor/3(DCM) -> Wind and Resistance (Real)/2(DCM), mg/1(DCM), Log Acceration/1(DCM_be)  "CBN^T"
  mg/1(mg_(b)) -> Add2/2
  Translation of the Quadrotor/5(Ab) -> Log Acceration/2(A_b)
  [Euler_real] -> Translation of the Quadrotor/2(Euler)
  [angular_velocity] -> Translation of the Quadrotor/3("p, q , r")
  [Euler_real] -> Reshape6/1
  [angular_velocity] -> Reshape7/1
  Translation of the Quadrotor/2(Xe) -> Reshape5/1
  Mux1/1 -> x_whole_real/1
  M_b/1 -> Reshape2/1
  HIL in the Loop for Rotation/1("Euler_real ") -> [Euler_real]
  HIL in the Loop for Rotation/2(Angular Velocity Real) -> [angular_velocity]
  HIL in the Loop for Rotation/3(Euler IMU) -> Mux3/1
  HIL in the Loop for Rotation/4(Angular Velocity IMU) -> Mux3/2
  Mux3/1 -> "x_angular_IMU (x_Euler, Omega)"/1
  Wind and Resistance (Real)/1(F_wind_body) -> Add2/1
  Translation of the Quadrotor/4(Vb) -> Wind and Resistance (Real)/1(v_quadrotor_body)
  Reshape2/1 -> Add1/1
  Add1/1 -> HIL in the Loop for Rotation/2(M)
  Rotational Disturbance/1 -> M/1
  Mux2/1 -> [LOG_Output_real]
  Selector/1 -> Mux2/2
  [Euler_real] -> Selector/1
  [Euler_real] -> [LOG_TB_Angles]
  [angular_velocity] -> [LOG_TB_Angular_Velocities]

== system full_simulation_split_hil_new_connection/Reference System/Reference System ==
  command : Inport
  nu_hedge : Inport  Port=2
  Demux : Demux
  Demux1 : Demux
  LTI System Fifth Order : Subsystem  mask{den_ref=den_x_ref}
      mask prompts: den_ref "denominator of the transfer function"
  LTI System Fifth Order1 : Subsystem  mask{den_ref=den_y_ref}
      mask prompts: den_ref "denominator of the transfer function"
  LTI System Fifth Order2 : Subsystem  mask{den_ref=den_z_ref}
      mask prompts: den_ref "denominator of the transfer function"
  LTI System Third Order1 : Subsystem  mask{den_ref=den_psi_ref}
      mask prompts: den_ref "denominator of the transfer function"
  Mux : Mux
  Mux1 : Mux
  Mux2 : Mux
  nu : Outport
  y_ref : Outport  Port=2
  xi_ref : Outport  Port=3
  tag scope: LOG_External_Dynamics_Ref_Vector=global, LOG_Reference=global
  wires:
  command/1 -> Demux/1
  Demux/1 -> LTI System Fifth Order/1(u)
  Demux/2 -> LTI System Fifth Order1/1(u)
  Demux/3 -> LTI System Fifth Order2/1(u)
  Demux/4 -> LTI System Third Order1/1(u)
  LTI System Fifth Order/2(nu) -> Mux/1
  LTI System Fifth Order1/2(nu) -> Mux/2
  LTI System Fifth Order2/2(nu) -> Mux/3
  LTI System Third Order1/2(nu) -> Mux/4
  Mux/1 -> nu/1
  nu_hedge/1 -> Demux1/1
  Demux1/1 -> LTI System Fifth Order/2(nu_hedge)
  Demux1/2 -> LTI System Fifth Order1/2(nu_hedge)
  Demux1/3 -> LTI System Fifth Order2/2(nu_hedge)
  Demux1/4 -> LTI System Third Order1/2(nu_hedge)
  Mux1/1 -> y_ref/1, [LOG_Reference]
  Mux2/1 -> xi_ref/1, [LOG_External_Dynamics_Ref_Vector]
  LTI System Fifth Order/1(y_ref) -> Mux1/1
  LTI System Fifth Order1/1(y_ref) -> Mux1/2
  LTI System Fifth Order2/1(y_ref) -> Mux1/3
  LTI System Third Order1/1(y_ref) -> Mux1/4
  LTI System Fifth Order/3(ref_sig) -> Mux2/1
  LTI System Fifth Order1/3(ref_sig) -> Mux2/2
  LTI System Fifth Order2/3(ref_sig) -> Mux2/3
  LTI System Third Order1/3(ref_sig) -> Mux2/4

== system full_simulation_split_hil_new_connection/Dynamic Extension for the Actuator Signal/Limit xi1/Detect Rise Nonnegative ==
  note: Edge
  note: U(k)
  U : Inport
  Delay Input1 : UnitDelay  Description=Store in Global RAM  DisableCoverage=on  X0=vinit  SampleTime=-1
  FixPt Relational Operator : RelationalOperator  Operator=>  OutDataTypeStr=uint(8)  ZeroCross=off
  Y : Outport  InitialOutput=0
  wires:
  FixPt Relational Operator/1 -> Y/1
  Delay Input1/1 -> FixPt Relational Operator/2  "U(k-1)"
  U/1 -> FixPt Relational Operator/1, Delay Input1/1  "U(k)"

== system full_simulation_split_hil_new_connection/Quadrotor Dynamics with HIL1/Sensor Model/Noise ==
  In1 : Inport
  Add2 : Sum
  Mux2 : Mux  Inputs=3
  Noise x : RandomNumber  Variance=std_dev_x^2  Seed=seed_x  SampleTime=0
  Noise x1 : RandomNumber  Variance=std_dev_y^2  Seed=seed_y  SampleTime=0
  Noise x2 : RandomNumber  Variance=std_dev_z^2  Seed=seed_z  SampleTime=0
  Pulse Generator1 : DiscretePulseGenerator  PulseType=Time based  Period=sample_time_noise_x  PulseWidth=50
  Pulse Generator2 : DiscretePulseGenerator  PulseType=Time based  Period=sample_time_noise_y  PulseWidth=50
  Pulse Generator3 : DiscretePulseGenerator  PulseType=Time based  Period=sample_time_noise_z  PulseWidth=50
  Reshape4 : Reshape  OutputDimensionality=Column vector (2-D)  OutputDimensions=[1:3]
  Sample and Hold : dspsigops/Sample and Hold  trig=Rising edge  initCond=0  latchinput=off
  Sample and Hold1 : dspsigops/Sample and Hold  trig=Rising edge  initCond=0  latchinput=off
  Sample and Hold2 : dspsigops/Sample and Hold  trig=Rising edge  initCond=0  latchinput=off
  Out1 : Outport
  wires:
  In1/1 -> Reshape4/1
  Noise x/1 -> Sample and Hold/1
  Noise x1/1 -> Sample and Hold1/1
  Noise x2/1 -> Sample and Hold2/1
  Mux2/1 -> Add2/2
  Add2/1 -> Out1/1
  Reshape4/1 -> Add2/1
  Sample and Hold/1 -> Mux2/1
  Sample and Hold1/1 -> Mux2/2
  Sample and Hold2/1 -> Mux2/3
  Pulse Generator1/1 -> Sample and Hold/Trigger
  Pulse Generator2/1 -> Sample and Hold1/Trigger
  Pulse Generator3/1 -> Sample and Hold2/Trigger

== system full_simulation_split_hil_new_connection/Quadrotor Dynamics with HIL1/Sensor Model/Noise1 ==
  In1 : Inport
  Add2 : Sum
  Mux2 : Mux  Inputs=3
  Noise x : RandomNumber  Variance=std_dev_xp^2  Seed=seed_xp  SampleTime=0
  Noise x1 : RandomNumber  Variance=std_dev_yp^2  Seed=seed_yp  SampleTime=0
  Noise x2 : RandomNumber  Variance=std_dev_zp^2  Seed=seed_zp  SampleTime=0
  Reshape4 : Reshape  OutputDimensionality=Column vector (2-D)  OutputDimensions=[1:3]
  Out1 : Outport
  wires:
  Reshape4/1 -> Add2/1
  Add2/1 -> Out1/1
  Mux2/1 -> Add2/2
  In1/1 -> Reshape4/1
  Noise x/1 -> Mux2/1
  Noise x1/1 -> Mux2/2
  Noise x2/1 -> Mux2/3

== system full_simulation_split_hil_new_connection/Quadrotor Dynamics with HIL1/Sensor Model/Noise2 ==
  In1 : Inport
  Add2 : Sum
  Noise x : RandomNumber  Variance=std_dev_psi^2  Seed=seed_psi  SampleTime=0
  Pulse Generator1 : DiscretePulseGenerator  PulseType=Time based  Period=sample_time_noise_psi  PulseWidth=50
  Reshape4 : Reshape  OutputDimensionality=Column vector (2-D)  OutputDimensions=[1:3]
  Sample and Hold : dspsigops/Sample and Hold  trig=Rising edge  initCond=0  latchinput=off
  Out1 : Outport
  wires:
  In1/1 -> Reshape4/1
  Add2/1 -> Out1/1
  Reshape4/1 -> Add2/1
  Noise x/1 -> Sample and Hold/1
  Pulse Generator1/1 -> Sample and Hold/Trigger
  Sample and Hold/1 -> Add2/2

== system full_simulation_split_hil_new_connection/Quadrotor Dynamics with HIL1/Simulated Reality/HIL in the Loop for Rotation ==
  note: Real: simulated reality, no noise
      | IMU: IMU from QR
  F_z : Inport
  M : Inport  Port=2
  Gain1 : Gain  Gain=-1/K_Mot_Force/4
  Moment to Voltage : Subsystem
  Saturation : Saturate  UpperLimit=PWM_MAX  LowerLimit=0
  Sum2 : Sum  Inputs=++|
  Test Rig : Subsystem
  Voltage to PWM : Gain  Gain=255/13
  "Euler_real " : Outport
  Angular Velocity Real : Outport  Port=2
  Euler IMU : Outport  Port=3
  Angular Velocity IMU : Outport  Port=4
  tag scope: LOG_Motor_Input_Vector=global
  wires:
  Moment to Voltage/1(U (Spannungen)) -> Sum2/2
  Sum2/1 -> Voltage to PWM/1, [LOG_Motor_Input_Vector]
  Voltage to PWM/1 -> Saturation/1
  Gain1/1 -> Sum2/1
  F_z/1 -> Gain1/1
  M/1 -> Moment to Voltage/1(U (Momente))
  Saturation/1 -> Test Rig/1(U as PWM)
  Test Rig/1("Euler_real ") -> "Euler_real "/1
  Test Rig/2(Angular Velocity Real) -> Angular Velocity Real/1
  Test Rig/3(Euler IMU) -> Euler IMU/1
  Test Rig/4(Angular Velocity IMU) -> Angular Velocity IMU/1

== system full_simulation_split_hil_new_connection/Quadrotor Dynamics with HIL1/Simulated Reality/Log Acceration ==
  DCM_be : Inport
  A_b : Inport  Port=2
  Divide1 : Product  Inputs=**  Multiplication=Matrix(*)
  Transpose : dspmtrx3/Transpose  Hermitian=off  overflowFlag=off
  tag scope: LOG_Accelerations=global
  wires:
  Divide1/1 -> [LOG_Accelerations]
  Transpose/1 -> Divide1/1
  DCM_be/1 -> Transpose/1
  A_b/1 -> Divide1/2

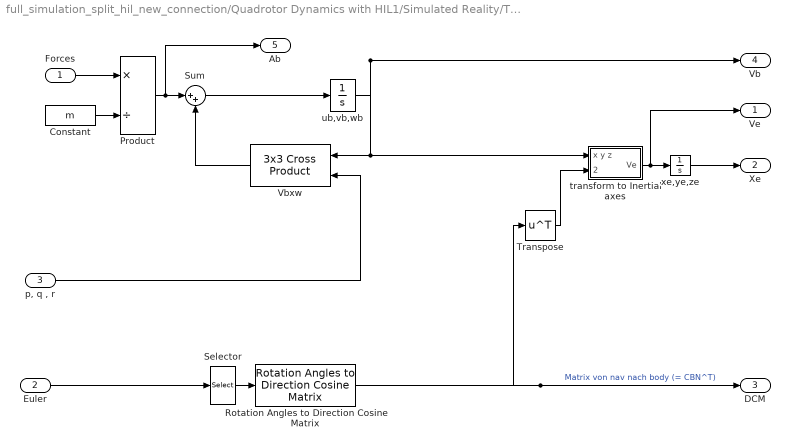
== system full_simulation_split_hil_new_connection/Quadrotor Dynamics with HIL1/Simulated Reality/Translation of the Quadrotor ==
  Forces : Inport
  Euler : Inport  Port=2
  "p, q , r" : Inport  Port=3
  Constant : Constant  Value=m  OutDataTypeStr=Inherit: Inherit via back propagation
  Product : Product  Inputs=*/  SaturateOnIntegerOverflow=on  OutDataTypeStr=Inherit: Same as first input
  Rotation Angles to Direction Cosine Matrix : aerolibtransform2/Rotation Angles to Direction Cosine Matrix  rotationOrder=ZYX
  Selector : Selector  InputPortWidth=3  IndexOptions=Index vector (dialog)  Indices=[3 2 1]  OutputSizes=1
  Sum : Sum  Inputs=|++  SaturateOnIntegerOverflow=on
  Transpose : Math  Operator=transpose  SaturateOnIntegerOverflow=on
  Vbxw : aerolibutil/3x3 Cross Product
  "transform to Inertial axes " : Subsystem
      mask Type: Vector Transformation
      mask Display: disp('L_EB')
  ub,vb,wb : Integrator
  xe,ye,ze : Integrator
  Ve : Outport
  Xe : Outport  Port=2
  DCM : Outport  Port=3
  Vb : Outport  Port=4
  Ab : Outport  Port=5
  wires:
  Constant/1 -> Product/2
  Transpose/1 -> "transform to Inertial axes "/2(transform coefficients)
  Product/1 -> Ab/1, Sum/1
  Forces/1 -> Product/1
  "transform to Inertial axes "/1(Ve) -> xe,ye,ze/1, Ve/1
  xe,ye,ze/1 -> Xe/1
  Sum/1 -> ub,vb,wb/1
  ub,vb,wb/1 -> Vbxw/1, "transform to Inertial axes "/1(x y z), Vb/1
  Vbxw/1 -> Sum/2
  Selector/1 -> Rotation Angles to Direction Cosine Matrix/1
  Euler/1 -> Selector/1
  "p, q , r"/1 -> Vbxw/2
  Rotation Angles to Direction Cosine Matrix/1 -> DCM/1, Transpose/1  "Matrix von nav nach body (= CBN^T)"

== system full_simulation_split_hil_new_connection/Quadrotor Dynamics with HIL1/Simulated Reality/Vertical Force Model ==
  F_z : Inport
  F_z to F(b) : Gain  Gain=[0; 0; Fz_gain]
  F_b : Outport
  wires:
  F_z/1 -> F_z to F(b)/1
  F_z to F(b)/1 -> F_b/1

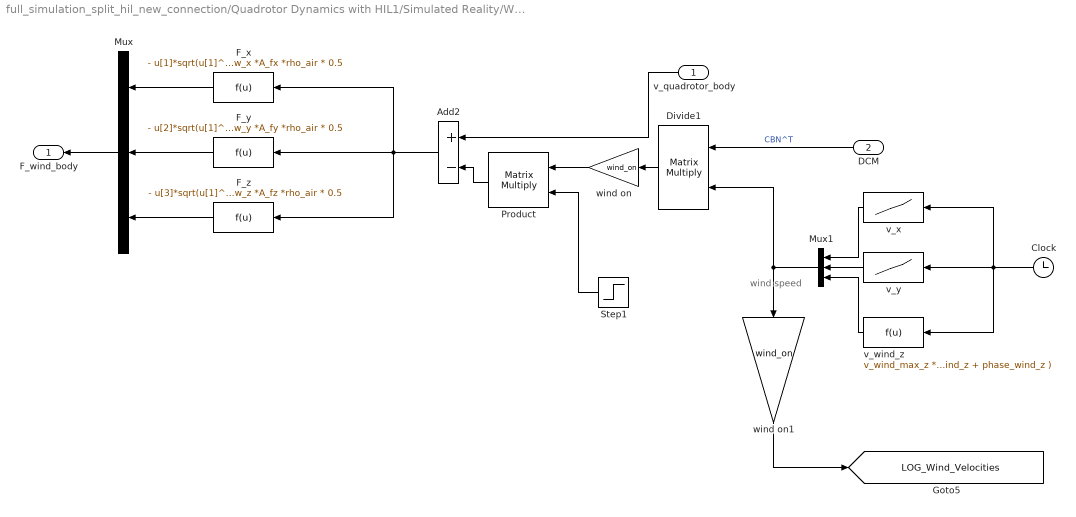
== system full_simulation_split_hil_new_connection/Quadrotor Dynamics with HIL1/Simulated Reality/Wind and Resistance (Real) ==
  note: wind speed
  v_quadrotor_body : Inport
  DCM : Inport  Port=2
  Add2 : Sum  Inputs=+-
  Clock : Clock
  Divide1 : Product  Inputs=**  Multiplication=Matrix(*)
  F_x : Fcn  Expr=- u[1]*sqrt(u[1]^2+u[2]^2+u[3]^2) *cw_x *A_fx *rho_air * 0.5
  F_y : Fcn  Expr=- u[2]*sqrt(u[1]^2+u[2]^2+u[3]^2) *cw_y *A_fy *rho_air * 0.5
  F_z : Fcn  Expr=- u[3]*sqrt(u[1]^2+u[2]^2+u[3]^2) *cw_z *A_fz *rho_air * 0.5
  Mux : Mux  Inputs=3
  Mux1 : Mux  Inputs=3
  Product : Product  Multiplication=Matrix(*)  RndMeth=Zero
  Step1 : Step  Time=15  SampleTime=0
  v_wind_z : Fcn  Expr=v_wind_max_z * sin(u[1] /T_wind_z + phase_wind_z )
  v_x : Lookup  InputValues=T_wind_fine  Table=v_wind_x_fine  LookUpMeth=Interpolation-Use End Values
  v_y : Lookup  InputValues=T_wind_fine  Table=v_wind_y_fine  LookUpMeth=Interpolation-Use End Values
  wind on : Gain  Gain=wind_on
  wind on1 : Gain  Gain=wind_on
  F_wind_body : Outport
  tag scope: LOG_Wind_Velocities=global
  wires:
  DCM/1 -> Divide1/1  "CBN^T"
  F_x/1 -> Mux/1
  F_y/1 -> Mux/2
  F_z/1 -> Mux/3
  v_x/1 -> Mux1/1
  v_y/1 -> Mux1/2
  v_wind_z/1 -> Mux1/3
  Clock/1 -> v_wind_z/1, v_x/1, v_y/1
  Mux1/1 -> Divide1/2, wind on1/1
  v_quadrotor_body/1 -> Add2/1
  Mux/1 -> F_wind_body/1
  Divide1/1 -> wind on/1
  Add2/1 -> F_y/1, F_z/1, F_x/1
  wind on1/1 -> [LOG_Wind_Velocities]
  Product/1 -> Add2/2
  wind on/1 -> Product/1
  Step1/1 -> Product/2

== system full_simulation_split_hil_new_connection/Quadrotor Dynamics with HIL1/Simulated Reality/mg ==
  DCM : Inport
  Constant2 : Constant  Value=[0; 0; m_real*g]
  Divide1 : Product  Inputs=**  Multiplication=Matrix(*)
  Reshape1 : Reshape  OutputDimensions=[1:3]
  mg_(b) : Outport
  wires:
  DCM/1 -> Divide1/1
  Divide1/1 -> Reshape1/1
  Constant2/1 -> Divide1/2
  Reshape1/1 -> mg_(b)/1

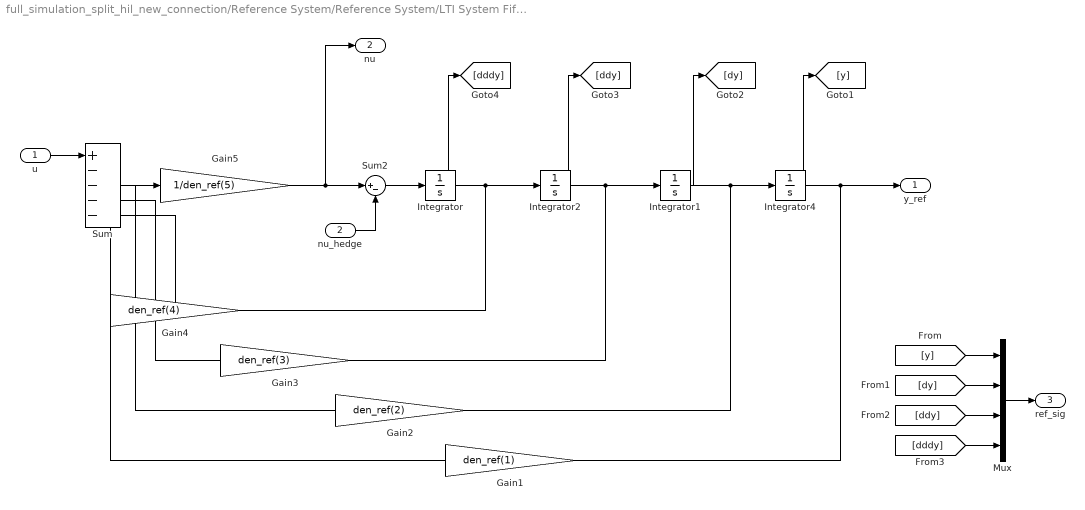
== system full_simulation_split_hil_new_connection/Reference System/Reference System/LTI System Fifth Order ==
  u : Inport
  nu_hedge : Inport  Port=2
  Gain1 : Gain  Gain=den_ref(1)
  Gain2 : Gain  Gain=den_ref(2)
  Gain3 : Gain  Gain=den_ref(3)
  Gain4 : Gain  Gain=den_ref(4)
  Gain5 : Gain  Gain=1/den_ref(5)
  Integrator{,1..2,4} (4 alike) : Integrator
  Mux : Mux
  Sum : Sum  Inputs=+----
  Sum2 : Sum  Inputs=|+-
  y_ref : Outport
  nu : Outport  Port=2
  ref_sig : Outport  Port=3
  wires:
  Mux/1 -> ref_sig/1
  [dddy] -> Mux/4
  [ddy] -> Mux/3
  [dy] -> Mux/2
  [y] -> Mux/1
  nu_hedge/1 -> Sum2/2
  u/1 -> Sum/1
  Sum2/1 -> Integrator/1
  Gain5/1 -> nu/1, Sum2/1
  Gain4/1 -> Sum/5
  Gain3/1 -> Sum/4
  Gain2/1 -> Sum/3
  Gain1/1 -> Sum/2
  Integrator4/1 -> [y], y_ref/1, Gain1/1
  Sum/1 -> Gain5/1
  Integrator1/1 -> [dy], Gain2/1, Integrator4/1
  Integrator2/1 -> [ddy], Gain3/1, Integrator1/1
  Integrator/1 -> [dddy], Gain4/1, Integrator2/1

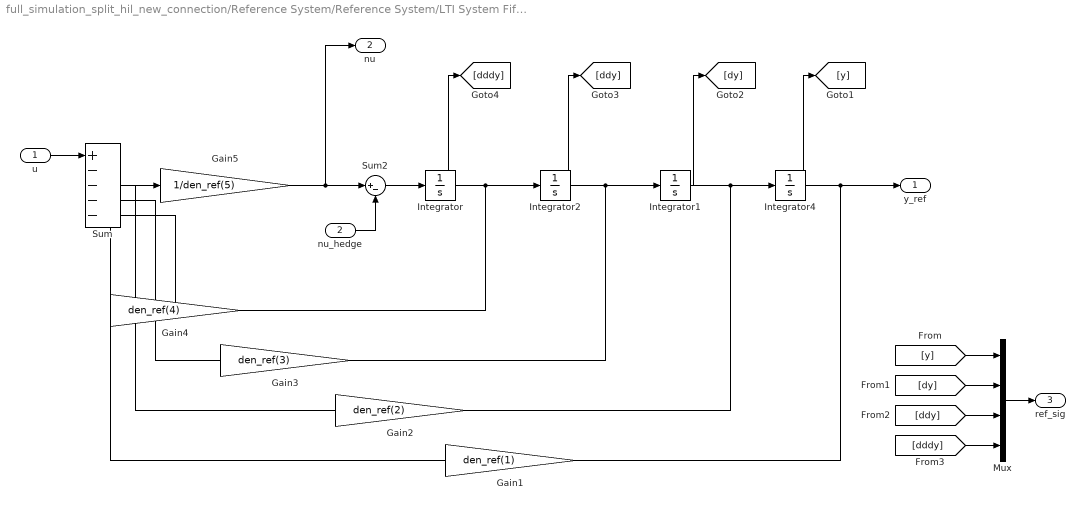
== system full_simulation_split_hil_new_connection/Reference System/Reference System/LTI System Fifth Order1 ==
  u : Inport
  nu_hedge : Inport  Port=2
  Gain1 : Gain  Gain=den_ref(1)
  Gain2 : Gain  Gain=den_ref(2)
  Gain3 : Gain  Gain=den_ref(3)
  Gain4 : Gain  Gain=den_ref(4)
  Gain5 : Gain  Gain=1/den_ref(5)
  Integrator{,1..2,4} (4 alike) : Integrator
  Mux : Mux
  Sum : Sum  Inputs=+----
  Sum2 : Sum  Inputs=|+-
  y_ref : Outport
  nu : Outport  Port=2
  ref_sig : Outport  Port=3
  wires:
  Integrator/1 -> Integrator2/1, Gain4/1, [dddy]
  Integrator2/1 -> Integrator1/1, Gain3/1, [ddy]
  Integrator1/1 -> Integrator4/1, Gain2/1, [dy]
  Sum/1 -> Gain5/1
  Integrator4/1 -> Gain1/1, y_ref/1, [y]
  Gain1/1 -> Sum/2
  Gain2/1 -> Sum/3
  Gain3/1 -> Sum/4
  Gain4/1 -> Sum/5
  Gain5/1 -> Sum2/1, nu/1
  Sum2/1 -> Integrator/1
  u/1 -> Sum/1
  nu_hedge/1 -> Sum2/2
  [y] -> Mux/1
  [dy] -> Mux/2
  [ddy] -> Mux/3
  [dddy] -> Mux/4
  Mux/1 -> ref_sig/1

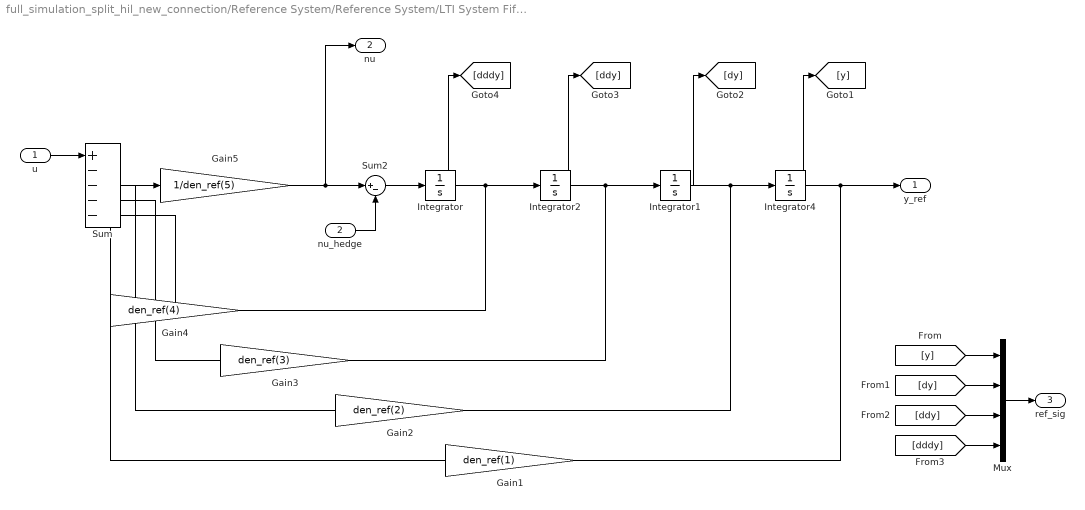
== system full_simulation_split_hil_new_connection/Reference System/Reference System/LTI System Fifth Order2 ==
  u : Inport
  nu_hedge : Inport  Port=2
  Gain1 : Gain  Gain=den_ref(1)
  Gain2 : Gain  Gain=den_ref(2)
  Gain3 : Gain  Gain=den_ref(3)
  Gain4 : Gain  Gain=den_ref(4)
  Gain5 : Gain  Gain=1/den_ref(5)
  Integrator{,1..2,4} (4 alike) : Integrator
  Mux : Mux
  Sum : Sum  Inputs=+----
  Sum2 : Sum  Inputs=|+-
  y_ref : Outport
  nu : Outport  Port=2
  ref_sig : Outport  Port=3
  wires:
  Mux/1 -> ref_sig/1
  [dddy] -> Mux/4
  [ddy] -> Mux/3
  [dy] -> Mux/2
  [y] -> Mux/1
  nu_hedge/1 -> Sum2/2
  u/1 -> Sum/1
  Sum2/1 -> Integrator/1
  Gain5/1 -> nu/1, Sum2/1
  Gain4/1 -> Sum/5
  Gain3/1 -> Sum/4
  Gain2/1 -> Sum/3
  Gain1/1 -> Sum/2
  Integrator4/1 -> [y], y_ref/1, Gain1/1
  Sum/1 -> Gain5/1
  Integrator1/1 -> [dy], Gain2/1, Integrator4/1
  Integrator2/1 -> [ddy], Gain3/1, Integrator1/1
  Integrator/1 -> [dddy], Gain4/1, Integrator2/1

== system full_simulation_split_hil_new_connection/Reference System/Reference System/LTI System Third Order1 ==
  u : Inport
  nu_hedge : Inport  Port=2
  Gain3 : Gain  Gain=den_ref(1)
  Gain4 : Gain  Gain=den_ref(2)
  Gain5 : Gain  Gain=1/den_ref(3)
  Integrator : Integrator
  Integrator2 : Integrator
  Mux : Mux  Inputs=2
  Sum : Sum  Inputs=+--
  Sum2 : Sum  Inputs=|+-
  y_ref : Outport
  nu : Outport  Port=2
  ref_sig : Outport  Port=3
  wires:
  Integrator/1 -> [dy], Integrator2/1, Gain4/1
  Integrator2/1 -> [y], y_ref/1, Gain3/1
  Sum/1 -> Gain5/1
  Gain3/1 -> Sum/2
  Gain4/1 -> Sum/3
  Gain5/1 -> Sum2/1, nu/1
  Sum2/1 -> Integrator/1
  u/1 -> Sum/1
  nu_hedge/1 -> Sum2/2
  [y] -> Mux/1
  [dy] -> Mux/2
  Mux/1 -> ref_sig/1

== system full_simulation_split_hil_new_connection/Quadrotor Dynamics with HIL1/Simulated Reality/HIL in the Loop for Rotation/Moment to Voltage ==
  U (Momente) : Inport
  Add : Sum  Inputs=+-
  Add1 : Sum  Inputs=-+
  Add2 : Sum
  Add3 : Sum  Inputs=--
  Demux : Demux  Outputs=3
  Gain1 : Gain  Gain=1/(2*K_Mot_Force*l)
  Gain2 : Gain  Gain=1/(2*K_Mot_Force*l)
  Gain3 : Gain  Gain=1/(K_Mot_Torque)/4
  Mux : Mux
  Mux1 : Mux  Inputs=3
  U (Spannungen) : Outport
  tag scope: LOG_delta_u=global
  wires:
  Demux/2 -> Gain2/1  "My"
  Add/1 -> Mux/1
  Add1/1 -> Mux/2
  Demux/1 -> Gain1/1  "Mx"
  Add2/1 -> Mux/4
  Gain1/1 -> Add1/1, Add2/1, Mux1/1
  Gain2/1 -> Add/1, Add3/1, Mux1/2
  Add3/1 -> Mux/3
  Gain3/1 -> Mux1/3, Add/2, Add1/2, Add3/2, Add2/2
  U (Momente)/1 -> Demux/1
  Mux/1 -> U (Spannungen)/1  "Spannungen"
  Demux/3 -> Gain3/1  "Mz"
  Mux1/1 -> [LOG_delta_u]
